simulink model "gm_three_in_adder"  (R2023a)
settings: Solver=FixedStepDiscrete  StartTime=0.0  StopTime=10.0  RelTol=1e-3
settings Model: Creator=szymadej  LastModifiedBy=szymadej
settings OptimizationCC: BlockReduction=off  ConditionallyExecuteInputs=off  DefaultParameterBehavior=Inlined  InheritOutputTypeSmallerThanSingle=on
settings DebuggingCC: AlgebraicLoopMsg=error  InheritedTsInSrcMsg=none  SingleTaskRateTransMsg=error  UnconnectedInputMsg=warning  UnconnectedOutputMsg=warning  UnconnectedLineMsg=warning
settings HardwareCC: ProdBitPerPointer=32  ProdBitPerSizeT=32  ProdBitPerPtrDiffT=32  ProdLargestAtomicFloat=None  ProdIntDivRoundTo=Undefined  ProdEndianess=Unspecified  ProdWordSize=32  ProdHWDeviceType=ASIC/FPGA->ASIC/FPGA  TargetBitPerLong=64  TargetBitPerPointer=64  TargetBitPerSizeT=64  TargetBitPerPtrDiffT=64  TargetLongLongMode=on  TargetIntDivRoundTo=Zero  TargetEndianess=LittleEndian  TargetWordSize=64  TargetHWDeviceType=Custom Processor->MATLAB Host Computer  ProdEqTarget=off

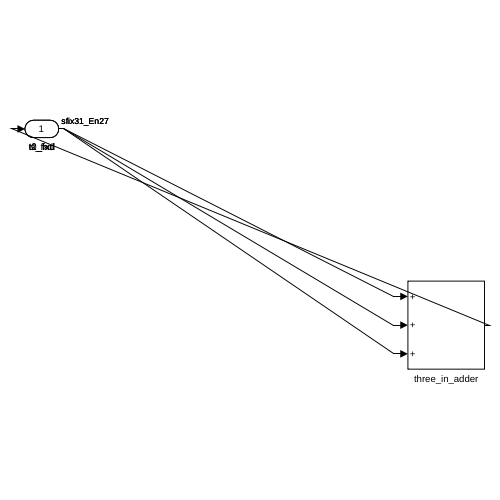
[thumbnail: Simulink's stored preview of the top-level diagram]
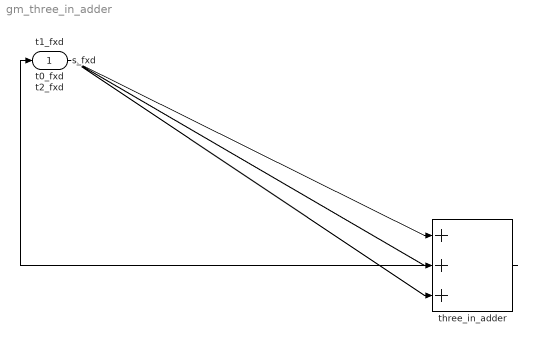
== system gm_three_in_adder ==
  t0_fxd : Inport  OutDataTypeStr=fixdt(1, 31, 27)  PortDimensions=1  SampleTime=0.2
  t1_fxd : Inport  Port=2  OutDataTypeStr=fixdt(1, 31, 27)  PortDimensions=1  SampleTime=0.2
  t2_fxd : Inport  Port=3  OutDataTypeStr=fixdt(1, 31, 27)  PortDimensions=1  SampleTime=0.2
  three_in_adder : Sum  Inputs=+++  OutDataTypeStr=fixdt(dt.s_fxd.s,dt.s_fxd.w,dt.s_fxd.f)
  s_fxd : Outport  SampleTime=0.2
  wires:
  t0_fxd/1 -> three_in_adder/1
  t1_fxd/1 -> three_in_adder/2
  t2_fxd/1 -> three_in_adder/3
  three_in_adder/1 -> s_fxd/1
